simulink model "counter_simple"  (R2014a)
settings: Solver=ode3  StartTime=0.0  StopTime=1000  FixedStep=1  RelTol=1e-3
libraries: hdlsllib x1
settings Model: Creator=Shiyu  LastModifiedBy=Shiyu

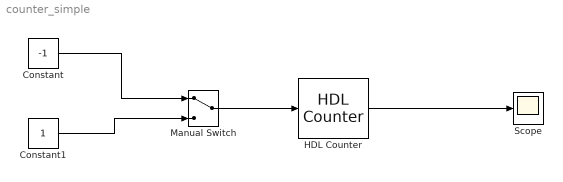
== system counter_simple ==
  Constant : Constant  Value=-1  OutDataTypeStr=boolean
  Constant1 : Constant  OutDataTypeStr=boolean
  HDL Counter : hdlsllib/HDL Operations/HDL Counter  CountType=Free running  CountInit=0  CountStep=1  CountMax=100  CountFromType=Initial value  CountFrom=0  CountResetPort=off  CountLoadPort=off  CountEnbPort=off  CountDirPort=on  CountDataType=Unsigned  CountWordLen=8  CountFracLen=0  CountSampTime=1
  Manual Switch : ManualSwitch
  Scope : Scope
  wires:
  Constant1/1 -> Manual Switch/2
  Constant/1 -> Manual Switch/1
  Manual Switch/1 -> HDL Counter/1
  HDL Counter/1 -> Scope/1
